simulink model "Fully_controlled_bridge_rectifier_18_04"  (R2020b)
settings: Solver=VariableStepAuto  StartTime=0.0  StopTime=.04  RelTol=1e-3
libraries: powerlib x10
settings Model: Creator=ADHIP  LastModifiedBy=ADHIP

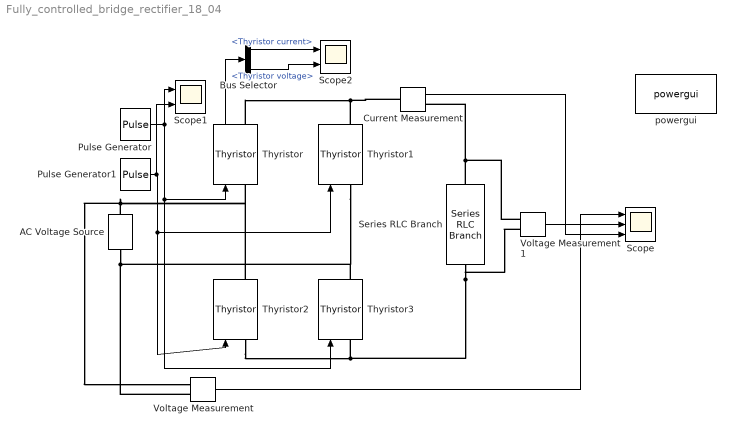
== system Fully_controlled_bridge_rectifier_18_04 ==
  AC Voltage Source : powerlib/Electrical Sources/AC Voltage Source  Amplitude=220*sqrt(2)  Phase=0  Frequency=50  SampleTime=0  Measurements=None  BusType=swing  Pref=10e3  Qref=0  Qmin=-inf  Qmax=+inf
  Bus Selector : BusSelector  OutputSignals=Thyristor current,Thyristor voltage
  Current Measurement : powerlib/Measurements/Current Measurement  PhasorSimulation=off  OutputType=Complex  PSBequivalent=0
  Pulse Generator : DiscretePulseGenerator  PulseType=Time based  Amplitude=50  Period=1/50  PulseWidth=5  PhaseDelay=0.02*15/360
  Pulse Generator1 : DiscretePulseGenerator  PulseType=Time based  Amplitude=50  Period=1/50  PulseWidth=5  PhaseDelay=0.02*195/360
  Scope : Scope  NumInputPorts=3
  Scope1 : Scope  NumInputPorts=2
  Scope2 : Scope  NumInputPorts=2
  Series RLC Branch : powerlib/Elements/Series RLC Branch  LConnTagsString=__new0  RConnTagsString=__new0  BranchType=RL  Resistance=1  Inductance=1e-3  SetiL0=off  InitialCurrent=0  Capacitance=1e-6  Setx0=off  InitialVoltage=0  Measurements=None
  Thyristor{,1..3} (4 alike) : powerlib/Power Electronics/Thyristor  Ron=0.001  Lon=0  Vf=0.8  IC=0  Rs=500  Cs=250e-9  Measurements=on
  Voltage Measurement : powerlib/Measurements/Voltage Measurement  PhasorSimulation=off  OutputType=Complex  PSBequivalent=0
  Voltage Measurement1 : powerlib/Measurements/Voltage Measurement  PhasorSimulation=off  OutputType=Complex  PSBequivalent=0
  powergui : powerlib/powergui  Priority=1  SimulationMode=Continuous  SampleTime=50e-6  frequency=60  Iterations=50  frequencyindice=50  Pbase=100e6  ErrMax=1e-4  UnitsV=kV  UnitsW=MW  buscounter=0  FunctionMessages=off  echomessages=off  EnableUseOfTLC=off  CurrentSourceSwitches=off  DisableSnubberDevices=off  DisableRonSwitches=off  DisableVfSwitches=off  DisplayEquations=off  AutomaticDiscreteSolvers=off  SolverType=Tustin/Backward Euler (TBE)  Interpol=off  ExternalGateDelay=off  methode=off  Ts=100  x0status=blocks  SPID=on  SwTol=0  HookPort=off  NonlinearTolerance=1e-4  nMaxIteration=100  ContinueOnMaxIteration=off  RestoreLinks=warning  ResistiveCurrentMeasurement=off  Frange=[0:2:500]  Ylog=off  Xlog=on  ShowGrid=off  save=off  variable=ZData  structure=0  ZoomFFT=off  StartTime=0.0  cycles=1  DisplayStyle=1  fundamental=60  FreqAxis=off  MaxFrequency=1000  frequencyindicesteady=1  RmsSteady=1  display=off
  wires:
  Bus Selector/2 -> Scope2/2  "<Thyristor voltage>"
  Current Measurement/1 -> Scope/3
  Voltage Measurement1/1 -> Scope/2
  Voltage Measurement/1 -> Scope/1
  Bus Selector/1 -> Scope2/1  "<Thyristor current>"
  Pulse Generator/1 -> Scope1/1, Thyristor/1, Thyristor3/1
  Pulse Generator1/1 -> Scope1/2, Thyristor1/1, Thyristor2/1
  Thyristor/1 -> Bus Selector/1
  connections:
  AC Voltage Source/LConn1 -- Voltage Measurement/LConn2 -- Thyristor3/RConn1 -- Thyristor1/LConn1
  AC Voltage Source/RConn1 -- Thyristor2/RConn1 -- Thyristor/LConn1 -- Voltage Measurement/LConn1
  Thyristor/RConn1 -- Current Measurement/LConn1 -- Thyristor1/RConn1
  Voltage Measurement1/LConn2 -- Series RLC Branch/RConn1 -- Thyristor2/LConn1 -- Thyristor3/LConn1
  Voltage Measurement1/LConn1 -- Series RLC Branch/LConn1 -- Current Measurement/RConn1
